simulink model "FullStateFeedbackEg_Sim"  (R2020a)
settings: Solver=FixedStepAuto  StartTime=0.0  StopTime=5  FixedStep=0.001  RelTol=1e-3
values from neighbouring files (symbols this model uses):
  D = 50    [FullStateFeedbackEg.m]
  K = 1000    [FullStateFeedbackEg.m]
  K1 = KC(1)    [FullStateFeedbackEg.m]
  K2 = KC(2)    [FullStateFeedbackEg.m]
  K3 = KC(3)    [FullStateFeedbackEg.m]
  K4 = KC(4)    [FullStateFeedbackEg.m]
  Ka = 1*2000    (= 2000)    [FullStateFeedbackEg.m]
  M1 = 1    [FullStateFeedbackEg.m]
  M2 = 2    [FullStateFeedbackEg.m]
settings Model: Creator=XShen  LastModifiedBy=Shen
settings DataIOCC: ReturnWorkspaceOutputs=off
settings DebuggingCC: ArithmeticOperatorsInVariantConditions=warning
settings SFSimCC: SimUseLocalCustomCode=off  CustomCodeUndefinedFunction=UseInterfaceOnly
settings RTWCC: RTWUseLocalCustomCode=off
settings CodeAppCC: StateflowObjectComments=on

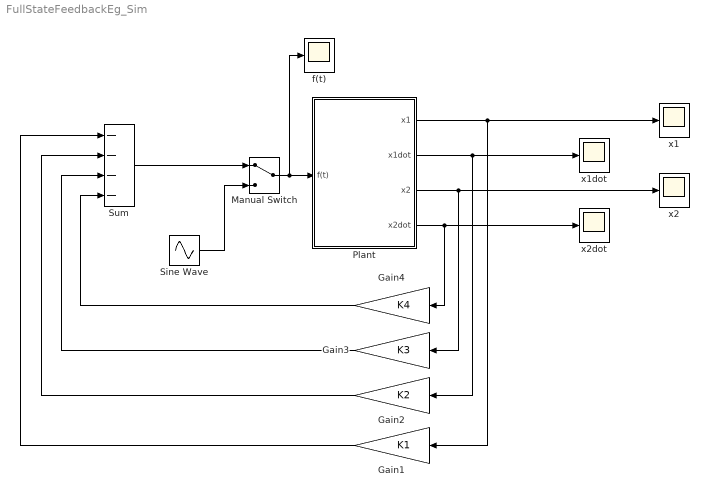
== system FullStateFeedbackEg_Sim ==
  Gain1 : Gain  Gain=K1
  Gain2 : Gain  Gain=K2
  Gain3 : Gain  Gain=K3
  Gain4 : Gain  Gain=K4
  Manual Switch : ManualSwitch
  "Plant " : Subsystem
  Sine Wave : Sin  Amplitude=0.1  SampleTime=0
  Sum : Sum  Inputs=----
  f(t) : Scope
  x1 : Scope
  x1dot : Scope
  x2 : Scope
  x2dot : Scope
  wires:
  "Plant "/1(x1) -> Gain1/1, x1/1
  "Plant "/4(x2dot) -> x2dot/1, Gain4/1
  "Plant "/3(x2) -> x2/1, Gain3/1
  "Plant "/2(x1dot) -> x1dot/1, Gain2/1
  Gain4/1 -> Sum/4
  Gain3/1 -> Sum/3
  Gain2/1 -> Sum/2
  Gain1/1 -> Sum/1
  Manual Switch/1 -> f(t)/1, "Plant "/1(f(t))
  Sum/1 -> Manual Switch/1
  Sine Wave/1 -> Manual Switch/2

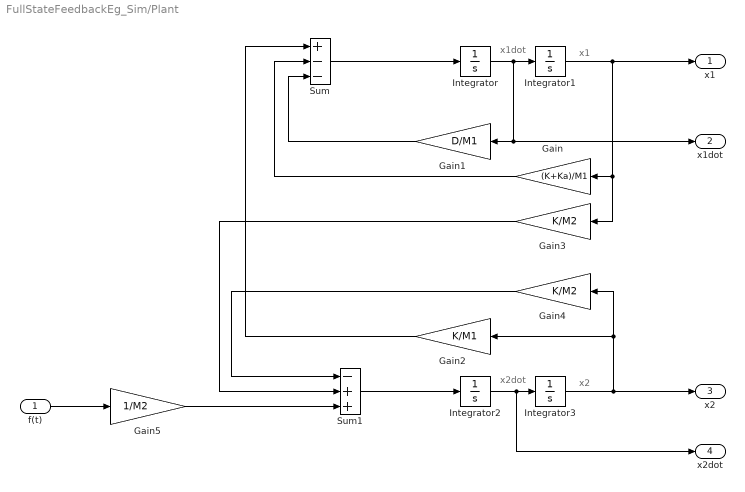
== system FullStateFeedbackEg_Sim/Plant  ==
  note: x1dot
  note: x1
  note: x2dot
  note: x2
  f(t) : Inport
  Gain : Gain  Gain=(K+Ka)/M1
  Gain1 : Gain  Gain=D/M1
  Gain2 : Gain  Gain=K/M1
  Gain3 : Gain  Gain=K/M2
  Gain4 : Gain  Gain=K/M2
  Gain5 : Gain  Gain=1/M2
  Integrator : Integrator
  Integrator1 : Integrator  InitialCondition=1
  Integrator2 : Integrator
  Integrator3 : Integrator
  Sum : Sum  Inputs=+--
  Sum1 : Sum  Inputs=-++
  x1 : Outport
  x1dot : Outport  Port=2
  x2 : Outport  Port=3
  x2dot : Outport  Port=4
  wires:
  Gain1/1 -> Sum/3
  f(t)/1 -> Gain5/1
  Gain/1 -> Sum/2
  Gain5/1 -> Sum1/3
  Gain4/1 -> Sum1/1
  Gain3/1 -> Sum1/2
  Gain2/1 -> Sum/1
  Integrator3/1 -> x2/1, Gain4/1, Gain2/1
  Sum/1 -> Integrator/1
  Integrator2/1 -> x2dot/1, Integrator3/1
  Sum1/1 -> Integrator2/1
  Integrator1/1 -> x1/1, Gain3/1, Gain/1
  Integrator/1 -> x1dot/1, Gain1/1, Integrator1/1
